simulink model "lab3es1ver7"  (R2021b)
settings: Solver=VariableStepAuto  StartTime=0.0  StopTime=3  RelTol=1e-3
values from neighbouring files (symbols this model uses):
  b = 1.0    (= 1)    [Lab4.m]
  g = 9.8    [Lab4.m]
  Ie = I+m*l^2    (= 0.026047)    [Lab4.m]
  k = 10    [Lab4.m]
  l = 0.305    [Lab4.m]
  m = 0.21    [Lab4.m]
  Me = m+M    (= 0.665)    [Lab4.m]
  x = [0, 0, pi/8, 0]    [Lab4.m]
settings Model: Creator=bonvoltnuovo  LastModifiedBy=bonaventur

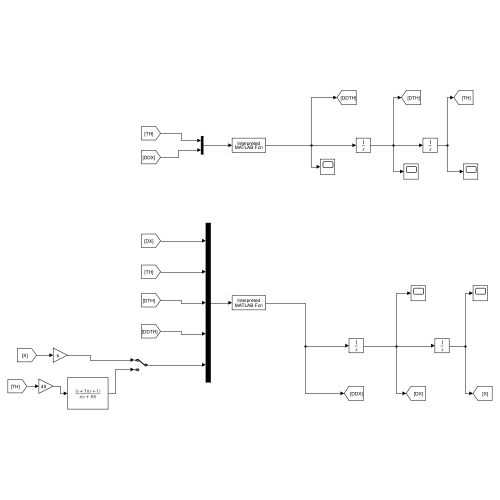
[thumbnail: Simulink's stored preview of the top-level diagram]
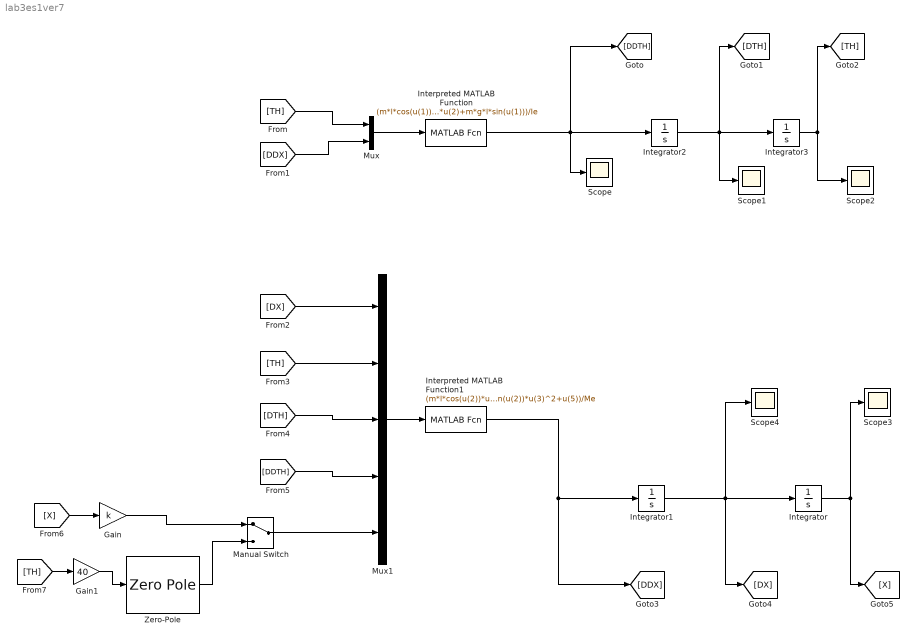
== system lab3es1ver7 ==
  Gain : Gain  Gain=k
  Gain1 : Gain  Gain=40
  Integrator : Integrator  InitialCondition=x(1)
  Integrator1 : Integrator  InitialCondition=x(2)
  Integrator2 : Integrator  InitialCondition=x(4)
  Integrator3 : Integrator  InitialCondition=x(3)
  Interpreted MATLAB Function : MATLABFcn  MATLABFcn=(m*l*cos(u(1))*u(2)+m*g*l*sin(u(1)))/Ie
  Interpreted MATLAB Function1 : MATLABFcn  MATLABFcn=(m*l*cos(u(2))*u(4)-b*u(1)-m*l*sin(u(2))*u(3)^2+u(5))/Me
  Manual Switch : ManualSwitch
  Mux : Mux  Inputs=2
  Mux1 : Mux  Inputs=5
  Scope{,1..4} (5 alike) : Scope
  Zero-Pole : ZeroPole  Zeros=[-3, -1]  Poles=[0 -10]
  wires:
  [DDX] -> Mux/2
  Mux/1 -> Interpreted MATLAB Function/1
  [TH] -> Mux/1
  Integrator2/1 -> Scope1/1, Integrator3/1, [DTH]
  Integrator3/1 -> Scope2/1, [TH]
  Integrator/1 -> [X], Scope3/1
  Integrator1/1 -> Scope4/1, Integrator/1, [DX]
  Interpreted MATLAB Function/1 -> Scope/1, [DDTH], Integrator2/1
  [DDTH] -> Mux1/4
  [TH] -> Mux1/2
  [DTH] -> Mux1/3
  [DX] -> Mux1/1
  Interpreted MATLAB Function1/1 -> Integrator1/1, [DDX]
  Mux1/1 -> Interpreted MATLAB Function1/1
  [X] -> Gain/1
  Gain/1 -> Manual Switch/1
  Manual Switch/1 -> Mux1/5
  Gain1/1 -> Zero-Pole/1
  Zero-Pole/1 -> Manual Switch/2
  [TH] -> Gain1/1
